simulink model "InfineonRacer"  (R2016b)
settings: Solver=FixedStepAuto  StartTime=0.0  StopTime=10.0  FixedStep=T_IR_Plant  MaxStep=0.1  RelTol=1e-3
undefined symbols (not defined in the file or in its folder): T_IR_Plant
settings Model: ModifiedByFormat=The MathWorks Inc.  Creator=The MathWorks Inc.  LastModifiedBy=The MathWorks Inc.
settings SolverCC: AutoInsertRateTranBlk=on
settings DataIOCC: LimitDataPoints=on  SaveFormat=Array
settings OptimizationCC: DefaultParameterBehavior=Inlined  ExpressionDepthLimit=2147483647  LifeSpan=1
settings DebuggingCC: UnderspecifiedInitializationDetection=Classic  MergeDetectMultiDrivingBlocksExec=none  SolverPrmCheckMsg=warning  FcnCallInpInsideContextMsg=warning  StateNameClashWarn=warning  SFUnexpectedBacktrackingDiag=warning  SFNoUnconditionalDefaultTransitionDiag=warning  SFExecutionAtInitializationDiag=none
settings HardwareCC: ProdBitPerPointer=32  ProdBitPerSizeT=32  ProdBitPerPtrDiffT=32  ProdLargestAtomicFloat=None  ProdIntDivRoundTo=Undefined  ProdEndianess=Unspecified  ProdWordSize=32  ProdHWDeviceType=32-bit Generic
settings ModelReferenceCC: PropagateSignalLabelsOutOfModel=off
settings GRTTargetCC: TargetLangStandard=C89/C90 (ANSI)  GeneratePreprocessorConditionals=Disable all  CombineOutputUpdateFcns=off  GRTInterface=on
settings ConfigComp: CovMetricSettings=dw  CovHtmlReporting=on  CovSaveCumulativeToWorkspaceVar=on  CovSaveSingleToWorkspaceVar=on  CovExternalEMLEnable=off

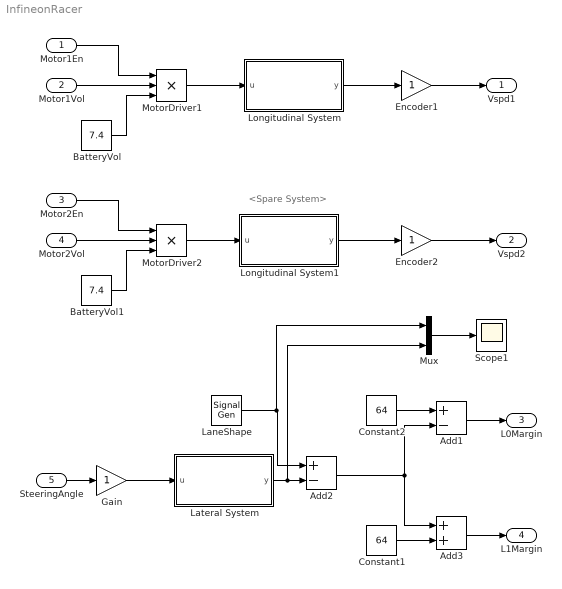
== system InfineonRacer ==
  note: <Spare System>
  Motor1En : Inport  SampleTime=T_IR_Plant
  Motor1Vol : Inport  Port=2  SampleTime=T_IR_Plant
  Motor2En : Inport  Port=3  SampleTime=T_IR_Plant
  Motor2Vol : Inport  Port=4  SampleTime=T_IR_Plant
  SteeringAngle : Inport  Port=5  SampleTime=T_IR_Plant
  Add1 : Sum  Inputs=+-
  Add2 : Sum  Inputs=+-
  Add3 : Sum
  BatteryVol : Constant  Value=7.4
  BatteryVol1 : Constant  Value=7.4
  Constant1 : Constant  Value=64
  Constant2 : Constant  Value=64
  Encoder1 : Gain
  Encoder2 : Gain
  Gain : Gain
  LaneShape : SignalGenerator  WaveForm=square  Amplitude=20  Frequency=0.5
  Lateral System : Subsystem  mask{wn=16, zeta=0.6}
      mask prompts: wn "Undamped natural frequency (wn, rad/s)"; zeta "Damping factor (zeta)"
  Longitudinal System : Subsystem  mask{wn=16, zeta=0.6}
      mask prompts: wn "Undamped natural frequency (wn, rad/s)"; zeta "Damping factor (zeta)"
  Longitudinal System1 : Subsystem  mask{wn=6, zeta=0.6}
      mask prompts: wn "Undamped natural frequency (wn, rad/s)"; zeta "Damping factor (zeta)"
  MotorDriver1 : Product  Inputs=3
  MotorDriver2 : Product  Inputs=3
  Mux : Mux  Inputs=2
  Scope1 : Scope
  Vspd1 : Outport
  Vspd2 : Outport  Port=2
  L0Margin : Outport  Port=3
  L1Margin : Outport  Port=4
  wires:
  MotorDriver1/1 -> Longitudinal System/1(u)
  Motor1En/1 -> MotorDriver1/1
  Motor1Vol/1 -> MotorDriver1/2
  BatteryVol/1 -> MotorDriver1/3
  MotorDriver2/1 -> Longitudinal System1/1(u)
  Motor2En/1 -> MotorDriver2/1
  Motor2Vol/1 -> MotorDriver2/2
  BatteryVol1/1 -> MotorDriver2/3
  Encoder1/1 -> Vspd1/1
  Encoder2/1 -> Vspd2/1
  Longitudinal System1/1(y) -> Encoder2/1
  Longitudinal System/1(y) -> Encoder1/1
  Add1/1 -> L0Margin/1
  LaneShape/1 -> Mux/1, Add2/1
  Lateral System/1(y) -> Mux/2, Add2/2
  Constant2/1 -> Add1/1
  Add2/1 -> Add3/1, Add1/2
  Add3/1 -> L1Margin/1
  Constant1/1 -> Add3/2
  SteeringAngle/1 -> Gain/1
  Gain/1 -> Lateral System/1(u)
  Mux/1 -> Scope1/1

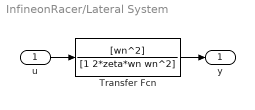
== system InfineonRacer/Lateral System ==
  u : Inport
  Transfer Fcn : TransferFcn  Numerator=[wn^2]  Denominator=[1 2*zeta*wn wn^2]
  y : Outport
  wires:
  Transfer Fcn/1 -> y/1
  u/1 -> Transfer Fcn/1

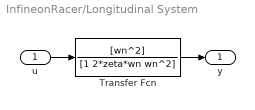
== system InfineonRacer/Longitudinal System ==
  u : Inport
  Transfer Fcn : TransferFcn  Numerator=[wn^2]  Denominator=[1 2*zeta*wn wn^2]
  y : Outport
  wires:
  Transfer Fcn/1 -> y/1
  u/1 -> Transfer Fcn/1

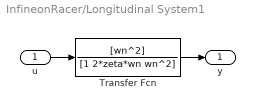
== system InfineonRacer/Longitudinal System1 ==
  u : Inport
  Transfer Fcn : TransferFcn  Numerator=[wn^2]  Denominator=[1 2*zeta*wn wn^2]
  y : Outport
  wires:
  Transfer Fcn/1 -> y/1
  u/1 -> Transfer Fcn/1
